simulink model "Challenge_Euler_Pos_state_space"  (R2024b)
settings: Solver=VariableStepAuto  StartTime=0.0  StopTime=10  RelTol=1e-3
values from neighbouring files (symbols this model uses):
  BackwardEuler_Gamma = (temp * Bo) * T    [Pos_state_space_code.m]
  BackwardEuler_H = Co * temp    [Pos_state_space_code.m]
  BackwardEuler_J = Do + Co * temp * Bo * T    [Pos_state_space_code.m]
  BackwardEuler_Phi = temp    [Pos_state_space_code.m]
  Exact_Gamma = inv(Ao) * ( Exact_Phi - I) * Bo    [Pos_state_space_code.m]
  Exact_H = Co    [Pos_state_space_code.m]
  Exact_J = Do    [Pos_state_space_code.m]
  Exact_Phi = expm(Ao*T)    [Pos_state_space_code.m]
  ForwardEuler_Gamma = Bo*T    [Pos_state_space_code.m]
  ForwardEuler_H = Co    [Pos_state_space_code.m]
  ForwardEuler_J = Do    [Pos_state_space_code.m]
  ForwardEuler_Phi = I + Ao*T    [Pos_state_space_code.m]
  K = place(A, B, CtrlPoles)    [Pos_state_space.m]    (also in Pos_state_space_code.m = acker(A,B,poles); code_ali.m = acker(A,B,poles); lab2_ali.m = acker(A,B,poles))
  Nu = Ans(3,1)    [Pos_state_space_code.m]    (also in code_ali.m; lab2_ali.m)
  Nx = Ans(1:2,1)    [Pos_state_space_code.m]    (also in code_ali.m; lab2_ali.m)
  T = 0.001*80    (= 0.08)    [Pos_state_space_code.m]
  Trapezoidal_Gamma = temp * Bo * sqrt(T)    [Pos_state_space_code.m]
  Trapezoidal_H = sqrt(T) * Co * temp    [Pos_state_space_code.m]
  Trapezoidal_J = Do + Co * temp * (Bo*T)/2    [Pos_state_space_code.m]
  Trapezoidal_Phi = (I + half_AT) * temp    [Pos_state_space_code.m]
undefined symbols (not defined in the file or in its folder): degs2rpm, rpm2rads
settings Model: Creator=UTENTE041019  LastModifiedBy=UTENTE041019

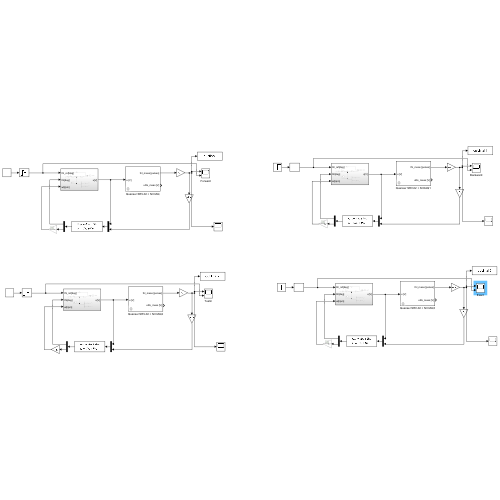
[thumbnail: Simulink's stored preview of the top-level diagram]
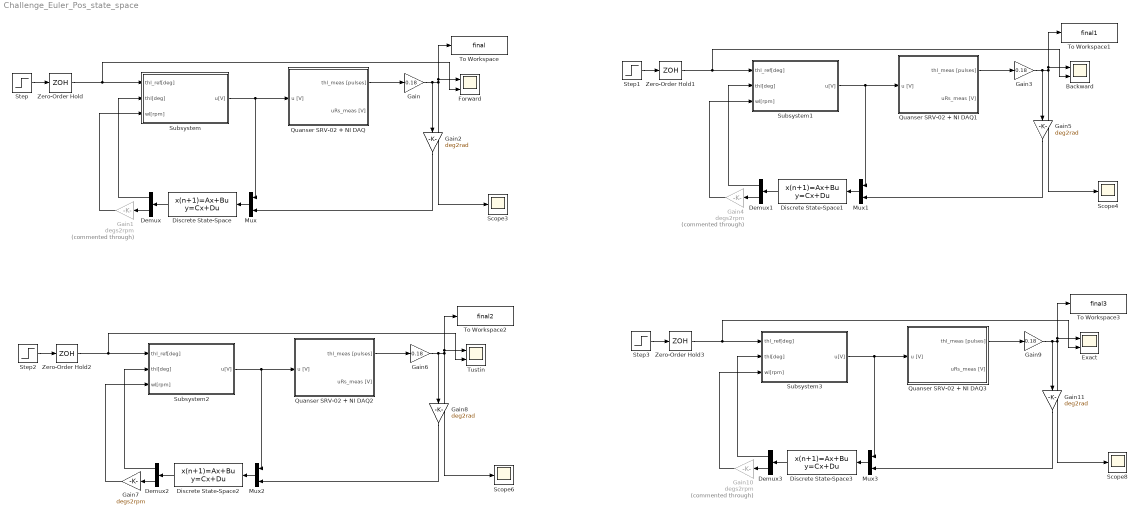
== system Challenge_Euler_Pos_state_space ==
  Backward : Scope  NumInputPorts=2
  Demux{,1..3} (4 alike) : Demux  Outputs=2
  Discrete State-Space : DiscreteStateSpace  A=ForwardEuler_Phi  B=ForwardEuler_Gamma  C=ForwardEuler_H  D=ForwardEuler_J  SampleTime=T
  Discrete State-Space1 : DiscreteStateSpace  A=BackwardEuler_Phi  B=BackwardEuler_Gamma  C=BackwardEuler_H  D=BackwardEuler_J  SampleTime=T
  Discrete State-Space2 : DiscreteStateSpace  A=Trapezoidal_Phi  B=Trapezoidal_Gamma  C=Trapezoidal_H  D=Trapezoidal_J  SampleTime=T
  Discrete State-Space3 : DiscreteStateSpace  A=Exact_Phi  B=Exact_Gamma  C=Exact_H  D=Exact_J  SampleTime=T
  Exact : Scope  NumInputPorts=2
  Forward : Scope  NumInputPorts=2
  Gain{,3,6,9} (4 alike) : Gain  Gain=0.18
  Gain1 : Gain  Commented=through  Gain=degs2rpm
  Gain10 : Gain  Commented=through  Gain=degs2rpm
  Gain{2,5,8,11} (4 alike) : Gain  Gain=deg2rad
  Gain4 : Gain  Commented=through  Gain=degs2rpm
  Gain7 : Gain  Gain=degs2rpm
  Mux{,1..3} (4 alike) : Mux  Inputs=2
  Quanser SRV-02 + NI DAQ : Subsystem  mask(Quanser SRV-02 (with inertial load) + NI DAQ){Ts=T, fricType=Coulomb + viscous}
      mask prompts: Ts "NI DAQ Sample Time:"; fricType "Friction model"
      mask help: Quanser SRV-02 (with inertial load) + NI DAQ model.
      mask init:
      | %%  Sensors data
      | 
      | %   shunt resistor
      | sens.curr.Rs = 0.5;                         %   resistance [Ohm]   
      | sens.curr.uRs_std = 0.01;                   %   voltage noise standard dev [V]                           
      | sens.curr.uRs_var = sens.curr.uRs_std^2;	%   voltage noise variance [V^2]
      | 
      | %   Hewlett-Packard HEDS-5540#A06 optical encoder
      | sens.enc.ppr = 500*4;                       %   pulses per rotation
      | sens.enc.pulse2deg = 360/sens.enc.ppr;      %   [pulses] -> [deg]
      | sens.enc.pulse2rad = 2*pi/sens.enc.ppr;     %   [pulses] -> [rad]
      | sens.enc.deg2pulse = sens.enc.ppr/360;      %   [deg] -> [pulses]
      | sens.enc.rad2pulse = sens.enc.ppr/2/pi;     %   [rad] -> [pulses]
      | 
      | 
      | %%  Data acquisition board (daq) data
      | 
      | %   NI PCI-6221 DAC data
      | daq.dac.bits = 16;                                  %   resolution (bits)
      | daq.dac.fs   = 10;                                  %   full scale 
      | daq.dac.q    = 2*daq.dac.fs/(2^daq.dac.bits-1);     %	quantization
      | 
      | %   NI PCI-6221 ADC data
      | daq.adc.bits = 16;                                  %   resolution (bits)
      | daq.adc.fs   = 10;                                  %   full scale (as set in SLDRT Analog Input block)
      | daq.adc.q    = 2*daq.adc.fs/(2^daq.adc.bits-1);     %   quantization
      mask Help:
      | Riccardo Antonello (antonello@dei.unipd.it)
      | 
      | April 24, 2020
      | 
      | Dept. of Information Engineering, University of Padova
      mask TypeOptions fricType: Coulomb + viscous | Karnopp
  Quanser SRV-02 + NI DAQ1 : Subsystem  mask(Quanser SRV-02 (with inertial load) + NI DAQ){Ts=T, fricType=Coulomb + viscous}
      mask prompts: Ts "NI DAQ Sample Time:"; fricType "Friction model"
      mask help: Quanser SRV-02 (with inertial load) + NI DAQ model.
      mask init: same as Challenge_Euler_Pos_state_space/Quanser SRV-02 + NI DAQ
      mask Help:
      | Riccardo Antonello (antonello@dei.unipd.it)
      | 
      | April 24, 2020
      | 
      | Dept. of Information Engineering, University of Padova
      mask TypeOptions fricType: Coulomb + viscous | Karnopp
  Quanser SRV-02 + NI DAQ2 : Subsystem  mask(Quanser SRV-02 (with inertial load) + NI DAQ){Ts=T, fricType=Coulomb + viscous}
      mask prompts: Ts "NI DAQ Sample Time:"; fricType "Friction model"
      mask help: Quanser SRV-02 (with inertial load) + NI DAQ model.
      mask init: same as Challenge_Euler_Pos_state_space/Quanser SRV-02 + NI DAQ
      mask Help:
      | Riccardo Antonello (antonello@dei.unipd.it)
      | 
      | April 24, 2020
      | 
      | Dept. of Information Engineering, University of Padova
      mask TypeOptions fricType: Coulomb + viscous | Karnopp
  Quanser SRV-02 + NI DAQ3 : Subsystem  mask(Quanser SRV-02 (with inertial load) + NI DAQ){Ts=T, fricType=Coulomb + viscous}
      mask prompts: Ts "NI DAQ Sample Time:"; fricType "Friction model"
      mask help: Quanser SRV-02 (with inertial load) + NI DAQ model.
      mask init: same as Challenge_Euler_Pos_state_space/Quanser SRV-02 + NI DAQ
      mask Help:
      | Riccardo Antonello (antonello@dei.unipd.it)
      | 
      | April 24, 2020
      | 
      | Dept. of Information Engineering, University of Padova
      mask TypeOptions fricType: Coulomb + viscous | Karnopp
  Scope{3..4,6,8} (4 alike) : Scope
  Step{,1..3} (4 alike) : Step  After=60  SampleTime=T
  Subsystem : Subsystem
  Subsystem1 : Subsystem
  Subsystem2 : Subsystem
  Subsystem3 : Subsystem
  To Workspace : ToWorkspace  VariableName=final  SaveFormat=Structure With Time  SampleTime=-1
  To Workspace1 : ToWorkspace  VariableName=final1  SaveFormat=Structure With Time  SampleTime=-1
  To Workspace2 : ToWorkspace  VariableName=final2  SaveFormat=Structure With Time  SampleTime=-1
  To Workspace3 : ToWorkspace  VariableName=final3  SaveFormat=Structure With Time  SampleTime=-1
  Tustin : Scope  NumInputPorts=2
  Zero-Order Hold{,1..3} (4 alike) : ZeroOrderHold  SampleTime=T
  wires:
  Quanser SRV-02 + NI DAQ/1(thl_meas [pulses]) -> Gain/1
  Gain/1 -> Gain2/1, To Workspace/1, Forward/1, Scope3/1
  Mux/1 -> Discrete State-Space/1
  Discrete State-Space/1 -> Demux/1
  Subsystem/1(u[V]) -> Mux/1, Quanser SRV-02 + NI DAQ/1(u [V])
  Demux/2 -> Gain1/1
  Gain1/1 -> Subsystem/3(wl[rpm])
  Demux/1 -> Subsystem/2(thl[deg])
  Step/1 -> Zero-Order Hold/1
  Zero-Order Hold/1 -> Forward/2, Subsystem/1(thl_ref[deg])
  Gain2/1 -> Mux/2
  Gain5/1 -> Mux1/2
  Discrete State-Space1/1 -> Demux1/1
  Gain4/1 -> Subsystem1/3(wl[rpm])
  Zero-Order Hold1/1 -> Backward/2, Subsystem1/1(thl_ref[deg])
  Demux1/2 -> Gain4/1
  Mux1/1 -> Discrete State-Space1/1
  Gain3/1 -> Gain5/1, To Workspace1/1, Backward/1, Scope4/1
  Quanser SRV-02 + NI DAQ1/1(thl_meas [pulses]) -> Gain3/1
  Subsystem1/1(u[V]) -> Mux1/1, Quanser SRV-02 + NI DAQ1/1(u [V])
  Demux1/1 -> Subsystem1/2(thl[deg])
  Step1/1 -> Zero-Order Hold1/1
  Gain8/1 -> Mux2/2
  Discrete State-Space2/1 -> Demux2/1
  Gain7/1 -> Subsystem2/3(wl[rpm])
  Zero-Order Hold2/1 -> Tustin/2, Subsystem2/1(thl_ref[deg])
  Demux2/2 -> Gain7/1
  Mux2/1 -> Discrete State-Space2/1
  Gain6/1 -> Gain8/1, To Workspace2/1, Tustin/1, Scope6/1
  Quanser SRV-02 + NI DAQ2/1(thl_meas [pulses]) -> Gain6/1
  Subsystem2/1(u[V]) -> Mux2/1, Quanser SRV-02 + NI DAQ2/1(u [V])
  Demux2/1 -> Subsystem2/2(thl[deg])
  Step2/1 -> Zero-Order Hold2/1
  Gain11/1 -> Mux3/2
  Discrete State-Space3/1 -> Demux3/1
  Gain10/1 -> Subsystem3/3(wl[rpm])
  Zero-Order Hold3/1 -> Exact/2, Subsystem3/1(thl_ref[deg])
  Demux3/2 -> Gain10/1
  Mux3/1 -> Discrete State-Space3/1
  Gain9/1 -> Gain11/1, To Workspace3/1, Exact/1, Scope8/1
  Quanser SRV-02 + NI DAQ3/1(thl_meas [pulses]) -> Gain9/1
  Subsystem3/1(u[V]) -> Mux3/1, Quanser SRV-02 + NI DAQ3/1(u [V])
  Demux3/1 -> Subsystem3/2(thl[deg])
  Step3/1 -> Zero-Order Hold3/1

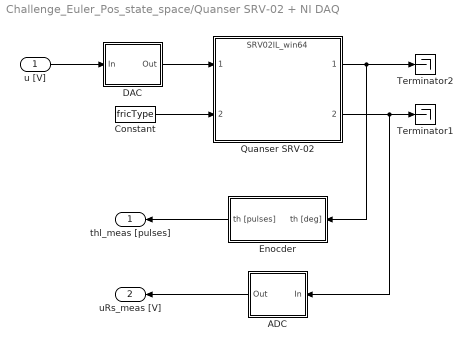
== system Challenge_Euler_Pos_state_space/Quanser SRV-02 + NI DAQ ==
  u [V] : Inport
  ADC : Subsystem
  Constant : Constant  Value=fricType
  DAC : Subsystem
  Enocder : Subsystem
  Quanser SRV-02 : ModelReference  ModelNameDialog=SRV02IL_win64.slxp  ModelReferenceVersion=1.44  CopyOfModelProtected=on
  Terminator1 : Terminator
  Terminator2 : Terminator
  thl_meas [pulses] : Outport
  uRs_meas [V] : Outport  Port=2
  wires:
  Enocder/1(th [pulses]) -> thl_meas [pulses]/1
  ADC/1(Out) -> uRs_meas [V]/1
  DAC/1(Out) -> Quanser SRV-02/1
  Quanser SRV-02/2 -> ADC/1(In), Terminator1/1
  u [V]/1 -> DAC/1(In)
  Quanser SRV-02/1 -> Enocder/1(th [deg]), Terminator2/1
  Constant/1 -> Quanser SRV-02/2

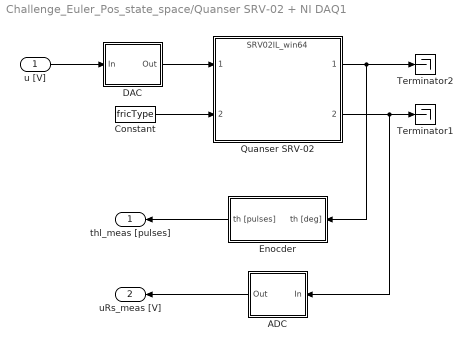
== system Challenge_Euler_Pos_state_space/Quanser SRV-02 + NI DAQ1 ==
  u [V] : Inport
  ADC : Subsystem
  Constant : Constant  Value=fricType
  DAC : Subsystem
  Enocder : Subsystem
  Quanser SRV-02 : ModelReference  ModelNameDialog=SRV02IL_win64.slxp  ModelReferenceVersion=1.44  CopyOfModelProtected=on
  Terminator1 : Terminator
  Terminator2 : Terminator
  thl_meas [pulses] : Outport
  uRs_meas [V] : Outport  Port=2
  wires:
  Enocder/1(th [pulses]) -> thl_meas [pulses]/1
  ADC/1(Out) -> uRs_meas [V]/1
  DAC/1(Out) -> Quanser SRV-02/1
  Quanser SRV-02/2 -> ADC/1(In), Terminator1/1
  u [V]/1 -> DAC/1(In)
  Quanser SRV-02/1 -> Enocder/1(th [deg]), Terminator2/1
  Constant/1 -> Quanser SRV-02/2

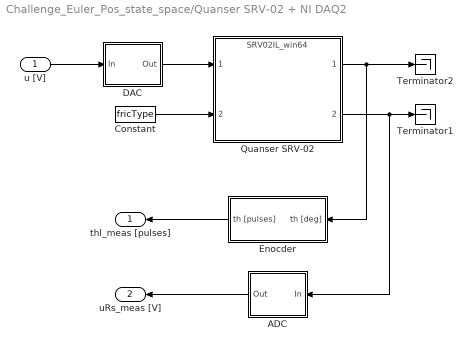
== system Challenge_Euler_Pos_state_space/Quanser SRV-02 + NI DAQ2 ==
  u [V] : Inport
  ADC : Subsystem
  Constant : Constant  Value=fricType
  DAC : Subsystem
  Enocder : Subsystem
  Quanser SRV-02 : ModelReference  ModelNameDialog=SRV02IL_win64.slxp  ModelReferenceVersion=1.44  CopyOfModelProtected=on
  Terminator1 : Terminator
  Terminator2 : Terminator
  thl_meas [pulses] : Outport
  uRs_meas [V] : Outport  Port=2
  wires:
  Enocder/1(th [pulses]) -> thl_meas [pulses]/1
  ADC/1(Out) -> uRs_meas [V]/1
  DAC/1(Out) -> Quanser SRV-02/1
  Quanser SRV-02/2 -> ADC/1(In), Terminator1/1
  u [V]/1 -> DAC/1(In)
  Quanser SRV-02/1 -> Enocder/1(th [deg]), Terminator2/1
  Constant/1 -> Quanser SRV-02/2

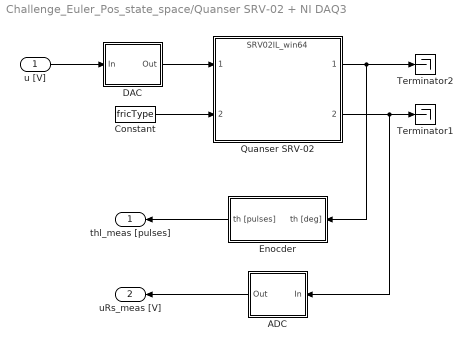
== system Challenge_Euler_Pos_state_space/Quanser SRV-02 + NI DAQ3 ==
  u [V] : Inport
  ADC : Subsystem
  Constant : Constant  Value=fricType
  DAC : Subsystem
  Enocder : Subsystem
  Quanser SRV-02 : ModelReference  ModelNameDialog=SRV02IL_win64.slxp  ModelReferenceVersion=1.44  CopyOfModelProtected=on
  Terminator1 : Terminator
  Terminator2 : Terminator
  thl_meas [pulses] : Outport
  uRs_meas [V] : Outport  Port=2
  wires:
  Enocder/1(th [pulses]) -> thl_meas [pulses]/1
  ADC/1(Out) -> uRs_meas [V]/1
  DAC/1(Out) -> Quanser SRV-02/1
  Quanser SRV-02/2 -> ADC/1(In), Terminator1/1
  u [V]/1 -> DAC/1(In)
  Quanser SRV-02/1 -> Enocder/1(th [deg]), Terminator2/1
  Constant/1 -> Quanser SRV-02/2

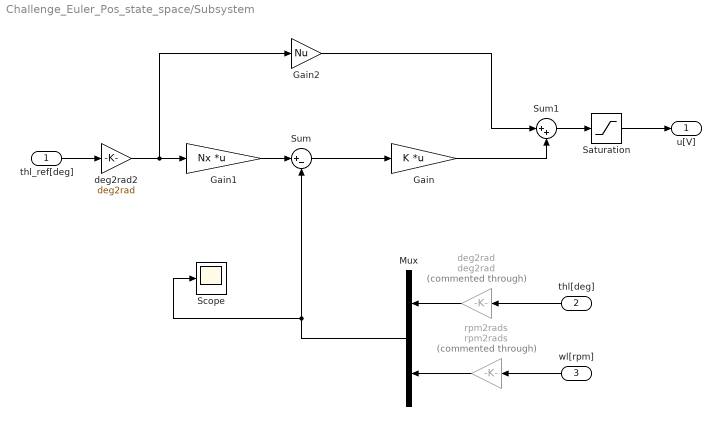
== system Challenge_Euler_Pos_state_space/Subsystem ==
  thl_ref[deg] : Inport
  thl[deg] : Inport  Port=2
  wl[rpm] : Inport  Port=3
  Gain : Gain  Gain=K  Multiplication=Matrix(K*u)
  Gain1 : Gain  Gain=Nx  Multiplication=Matrix(K*u)
  Gain2 : Gain  Gain=Nu
  Mux : Mux  Inputs=2
  Saturation : Saturate  UpperLimit=12  LowerLimit=-12
  Scope : Scope
  Sum : Sum  Inputs=|+-
  Sum1 : Sum  Inputs=|++
  deg2rad : Gain  Commented=through  Gain=deg2rad
  deg2rad2 : Gain  Gain=deg2rad
  rpm2rads : Gain  Commented=through  Gain=rpm2rads
  u[V] : Outport
  wires:
  thl[deg]/1 -> deg2rad/1
  wl[rpm]/1 -> rpm2rads/1
  deg2rad/1 -> Mux/1
  rpm2rads/1 -> Mux/2
  Mux/1 -> Sum/2, Scope/1
  Sum/1 -> Gain/1
  Gain1/1 -> Sum/1
  thl_ref[deg]/1 -> deg2rad2/1
  deg2rad2/1 -> Gain1/1, Gain2/1
  Gain2/1 -> Sum1/1
  Gain/1 -> Sum1/2
  Sum1/1 -> Saturation/1
  Saturation/1 -> u[V]/1

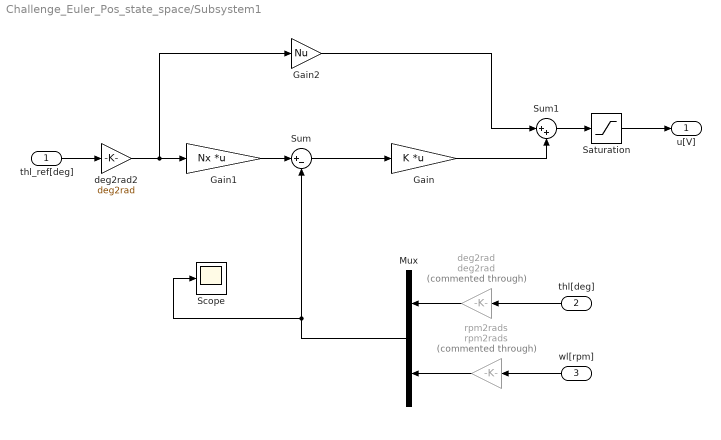
== system Challenge_Euler_Pos_state_space/Subsystem1 ==
  thl_ref[deg] : Inport
  thl[deg] : Inport  Port=2
  wl[rpm] : Inport  Port=3
  Gain : Gain  Gain=K  Multiplication=Matrix(K*u)
  Gain1 : Gain  Gain=Nx  Multiplication=Matrix(K*u)
  Gain2 : Gain  Gain=Nu
  Mux : Mux  Inputs=2
  Saturation : Saturate  UpperLimit=12  LowerLimit=-12
  Scope : Scope
  Sum : Sum  Inputs=|+-
  Sum1 : Sum  Inputs=|++
  deg2rad : Gain  Commented=through  Gain=deg2rad
  deg2rad2 : Gain  Gain=deg2rad
  rpm2rads : Gain  Commented=through  Gain=rpm2rads
  u[V] : Outport
  wires:
  thl[deg]/1 -> deg2rad/1
  wl[rpm]/1 -> rpm2rads/1
  deg2rad/1 -> Mux/1
  rpm2rads/1 -> Mux/2
  Mux/1 -> Sum/2, Scope/1
  Sum/1 -> Gain/1
  Gain1/1 -> Sum/1
  thl_ref[deg]/1 -> deg2rad2/1
  deg2rad2/1 -> Gain1/1, Gain2/1
  Gain2/1 -> Sum1/1
  Gain/1 -> Sum1/2
  Sum1/1 -> Saturation/1
  Saturation/1 -> u[V]/1

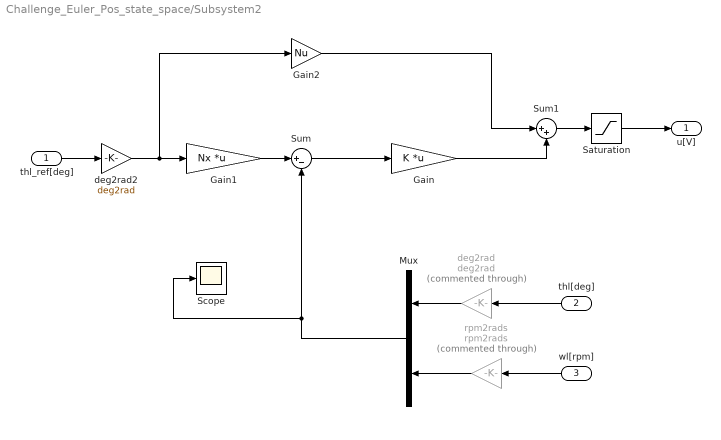
== system Challenge_Euler_Pos_state_space/Subsystem2 ==
  thl_ref[deg] : Inport
  thl[deg] : Inport  Port=2
  wl[rpm] : Inport  Port=3
  Gain : Gain  Gain=K  Multiplication=Matrix(K*u)
  Gain1 : Gain  Gain=Nx  Multiplication=Matrix(K*u)
  Gain2 : Gain  Gain=Nu
  Mux : Mux  Inputs=2
  Saturation : Saturate  UpperLimit=12  LowerLimit=-12
  Scope : Scope
  Sum : Sum  Inputs=|+-
  Sum1 : Sum  Inputs=|++
  deg2rad : Gain  Commented=through  Gain=deg2rad
  deg2rad2 : Gain  Gain=deg2rad
  rpm2rads : Gain  Commented=through  Gain=rpm2rads
  u[V] : Outport
  wires:
  thl[deg]/1 -> deg2rad/1
  wl[rpm]/1 -> rpm2rads/1
  deg2rad/1 -> Mux/1
  rpm2rads/1 -> Mux/2
  Mux/1 -> Sum/2, Scope/1
  Sum/1 -> Gain/1
  Gain1/1 -> Sum/1
  thl_ref[deg]/1 -> deg2rad2/1
  deg2rad2/1 -> Gain1/1, Gain2/1
  Gain2/1 -> Sum1/1
  Gain/1 -> Sum1/2
  Sum1/1 -> Saturation/1
  Saturation/1 -> u[V]/1

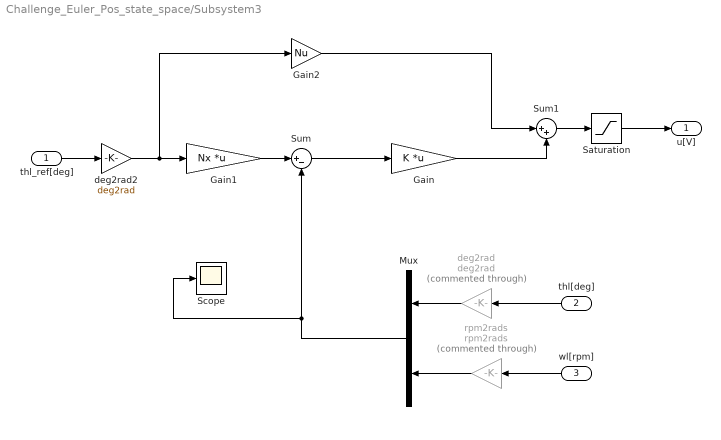
== system Challenge_Euler_Pos_state_space/Subsystem3 ==
  thl_ref[deg] : Inport
  thl[deg] : Inport  Port=2
  wl[rpm] : Inport  Port=3
  Gain : Gain  Gain=K  Multiplication=Matrix(K*u)
  Gain1 : Gain  Gain=Nx  Multiplication=Matrix(K*u)
  Gain2 : Gain  Gain=Nu
  Mux : Mux  Inputs=2
  Saturation : Saturate  UpperLimit=12  LowerLimit=-12
  Scope : Scope
  Sum : Sum  Inputs=|+-
  Sum1 : Sum  Inputs=|++
  deg2rad : Gain  Commented=through  Gain=deg2rad
  deg2rad2 : Gain  Gain=deg2rad
  rpm2rads : Gain  Commented=through  Gain=rpm2rads
  u[V] : Outport
  wires:
  thl[deg]/1 -> deg2rad/1
  wl[rpm]/1 -> rpm2rads/1
  deg2rad/1 -> Mux/1
  rpm2rads/1 -> Mux/2
  Mux/1 -> Sum/2, Scope/1
  Sum/1 -> Gain/1
  Gain1/1 -> Sum/1
  thl_ref[deg]/1 -> deg2rad2/1
  deg2rad2/1 -> Gain1/1, Gain2/1
  Gain2/1 -> Sum1/1
  Gain/1 -> Sum1/2
  Sum1/1 -> Saturation/1
  Saturation/1 -> u[V]/1

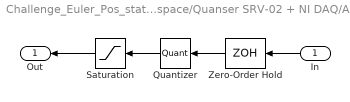
== system Challenge_Euler_Pos_state_space/Quanser SRV-02 + NI DAQ/ADC ==
  In : Inport
  Quantizer : Quantizer  QuantizationInterval=daq.adc.q
  Saturation : Saturate  UpperLimit=daq.adc.fs  LowerLimit=-daq.adc.fs
  Zero-Order Hold : ZeroOrderHold  SampleTime=Ts
  Out : Outport
  wires:
  Saturation/1 -> Out/1
  In/1 -> Zero-Order Hold/1
  Quantizer/1 -> Saturation/1
  Zero-Order Hold/1 -> Quantizer/1

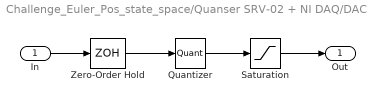
== system Challenge_Euler_Pos_state_space/Quanser SRV-02 + NI DAQ/DAC ==
  In : Inport
  Quantizer : Quantizer  QuantizationInterval=daq.dac.q
  Saturation : Saturate  UpperLimit=daq.dac.fs  LowerLimit=-daq.dac.fs
  Zero-Order Hold : ZeroOrderHold  SampleTime=Ts
  Out : Outport
  wires:
  Quantizer/1 -> Saturation/1
  In/1 -> Zero-Order Hold/1
  Zero-Order Hold/1 -> Quantizer/1
  Saturation/1 -> Out/1

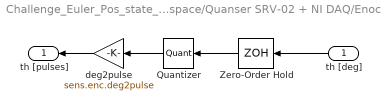
== system Challenge_Euler_Pos_state_space/Quanser SRV-02 + NI DAQ/Enocder ==
  th [deg] : Inport
  Quantizer : Quantizer  QuantizationInterval=sens.enc.pulse2deg
  Zero-Order Hold : ZeroOrderHold  SampleTime=Ts
  deg2pulse : Gain  Gain=sens.enc.deg2pulse
  th [pulses] : Outport
  wires:
  Quantizer/1 -> deg2pulse/1
  th [deg]/1 -> Zero-Order Hold/1
  Zero-Order Hold/1 -> Quantizer/1
  deg2pulse/1 -> th [pulses]/1

== system Challenge_Euler_Pos_state_space/Quanser SRV-02 + NI DAQ1/ADC ==
  In : Inport
  Quantizer : Quantizer  QuantizationInterval=daq.adc.q
  Saturation : Saturate  UpperLimit=daq.adc.fs  LowerLimit=-daq.adc.fs
  Zero-Order Hold : ZeroOrderHold  SampleTime=Ts
  Out : Outport
  wires:
  Saturation/1 -> Out/1
  In/1 -> Zero-Order Hold/1
  Quantizer/1 -> Saturation/1
  Zero-Order Hold/1 -> Quantizer/1

== system Challenge_Euler_Pos_state_space/Quanser SRV-02 + NI DAQ1/DAC ==
  In : Inport
  Quantizer : Quantizer  QuantizationInterval=daq.dac.q
  Saturation : Saturate  UpperLimit=daq.dac.fs  LowerLimit=-daq.dac.fs
  Zero-Order Hold : ZeroOrderHold  SampleTime=Ts
  Out : Outport
  wires:
  Quantizer/1 -> Saturation/1
  In/1 -> Zero-Order Hold/1
  Zero-Order Hold/1 -> Quantizer/1
  Saturation/1 -> Out/1

== system Challenge_Euler_Pos_state_space/Quanser SRV-02 + NI DAQ1/Enocder ==
  th [deg] : Inport
  Quantizer : Quantizer  QuantizationInterval=sens.enc.pulse2deg
  Zero-Order Hold : ZeroOrderHold  SampleTime=Ts
  deg2pulse : Gain  Gain=sens.enc.deg2pulse
  th [pulses] : Outport
  wires:
  Quantizer/1 -> deg2pulse/1
  th [deg]/1 -> Zero-Order Hold/1
  Zero-Order Hold/1 -> Quantizer/1
  deg2pulse/1 -> th [pulses]/1

== system Challenge_Euler_Pos_state_space/Quanser SRV-02 + NI DAQ2/ADC ==
  In : Inport
  Quantizer : Quantizer  QuantizationInterval=daq.adc.q
  Saturation : Saturate  UpperLimit=daq.adc.fs  LowerLimit=-daq.adc.fs
  Zero-Order Hold : ZeroOrderHold  SampleTime=Ts
  Out : Outport
  wires:
  Saturation/1 -> Out/1
  In/1 -> Zero-Order Hold/1
  Quantizer/1 -> Saturation/1
  Zero-Order Hold/1 -> Quantizer/1

== system Challenge_Euler_Pos_state_space/Quanser SRV-02 + NI DAQ2/DAC ==
  In : Inport
  Quantizer : Quantizer  QuantizationInterval=daq.dac.q
  Saturation : Saturate  UpperLimit=daq.dac.fs  LowerLimit=-daq.dac.fs
  Zero-Order Hold : ZeroOrderHold  SampleTime=Ts
  Out : Outport
  wires:
  Quantizer/1 -> Saturation/1
  In/1 -> Zero-Order Hold/1
  Zero-Order Hold/1 -> Quantizer/1
  Saturation/1 -> Out/1

== system Challenge_Euler_Pos_state_space/Quanser SRV-02 + NI DAQ2/Enocder ==
  th [deg] : Inport
  Quantizer : Quantizer  QuantizationInterval=sens.enc.pulse2deg
  Zero-Order Hold : ZeroOrderHold  SampleTime=Ts
  deg2pulse : Gain  Gain=sens.enc.deg2pulse
  th [pulses] : Outport
  wires:
  Quantizer/1 -> deg2pulse/1
  th [deg]/1 -> Zero-Order Hold/1
  Zero-Order Hold/1 -> Quantizer/1
  deg2pulse/1 -> th [pulses]/1

== system Challenge_Euler_Pos_state_space/Quanser SRV-02 + NI DAQ3/ADC ==
  In : Inport
  Quantizer : Quantizer  QuantizationInterval=daq.adc.q
  Saturation : Saturate  UpperLimit=daq.adc.fs  LowerLimit=-daq.adc.fs
  Zero-Order Hold : ZeroOrderHold  SampleTime=Ts
  Out : Outport
  wires:
  Saturation/1 -> Out/1
  In/1 -> Zero-Order Hold/1
  Quantizer/1 -> Saturation/1
  Zero-Order Hold/1 -> Quantizer/1

== system Challenge_Euler_Pos_state_space/Quanser SRV-02 + NI DAQ3/DAC ==
  In : Inport
  Quantizer : Quantizer  QuantizationInterval=daq.dac.q
  Saturation : Saturate  UpperLimit=daq.dac.fs  LowerLimit=-daq.dac.fs
  Zero-Order Hold : ZeroOrderHold  SampleTime=Ts
  Out : Outport
  wires:
  Quantizer/1 -> Saturation/1
  In/1 -> Zero-Order Hold/1
  Zero-Order Hold/1 -> Quantizer/1
  Saturation/1 -> Out/1

== system Challenge_Euler_Pos_state_space/Quanser SRV-02 + NI DAQ3/Enocder ==
  th [deg] : Inport
  Quantizer : Quantizer  QuantizationInterval=sens.enc.pulse2deg
  Zero-Order Hold : ZeroOrderHold  SampleTime=Ts
  deg2pulse : Gain  Gain=sens.enc.deg2pulse
  th [pulses] : Outport
  wires:
  Quantizer/1 -> deg2pulse/1
  th [deg]/1 -> Zero-Order Hold/1
  Zero-Order Hold/1 -> Quantizer/1
  deg2pulse/1 -> th [pulses]/1
